simulink model "LCSQ10"  (R2021a)
settings: Solver=VariableStepAuto  StartTime=0.0  StopTime=5  RelTol=1e-3
libraries: commchan3 x1
settings Model: Creator=M.M  LastModifiedBy=M.M

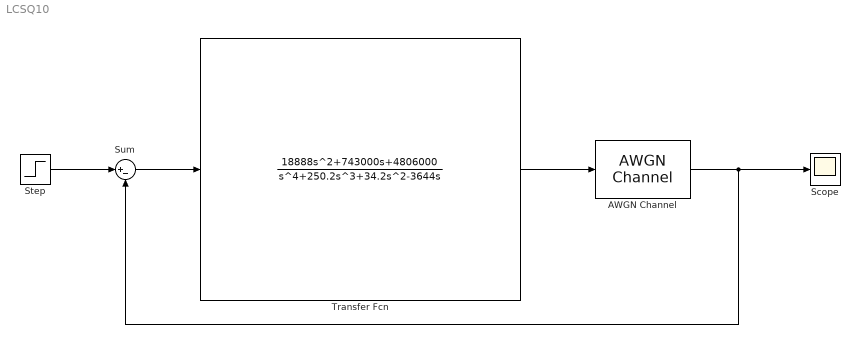
== system LCSQ10 ==
  AWGN Channel : commchan3/AWGN Channel  InputProcessing=Columns as channels (frame based)  seed=67  noiseMode="Signal to noise ratio  (SNR)"  EbNodB=10  EsNodB=10  SNRdB=10  bitsPerSym=1  Ps=0.001  Tsym=1  variance=1
  Scope : Scope
  Step : Step  Time=0  SampleTime=0
  Sum : Sum  Inputs=|+-
  Transfer Fcn : TransferFcn  Numerator=[0 0 18888 743000 4806000]  Denominator=[1 250.2 34.2 -3644 0]
  wires:
  Step/1 -> Sum/1
  Sum/1 -> Transfer Fcn/1
  Transfer Fcn/1 -> AWGN Channel/1
  AWGN Channel/1 -> Scope/1, Sum/2
